simulink model "EV_Modeling"  (R2024b)
(part 5 of 9)

  Signal Specification7/1 -> Divide36/1
  Divide38/1 -> [Motor_Power]
  Constant11/1 -> Switch1/3
  Integrator8/1 -> Position[m]/1, [Current_Position]
  Signal Specification8/1 -> Unit Conversion4/1
  From Workspace18/1 -> Divide33/2
  Add4/1 -> Gain17/1
  " Normalization"/3(Current_n) -> Mux2/3
  Divide22/1 -> Add15/2  "F_friction"
  Zero-Order Hold1/1 -> Extended Kalman Filter/2
  Mux2/1 -> LSTM/1(sequenceinput)
  Divide27/1 -> Add10/1  "Motor_Torque[N.m]"
  " Normalization"/1(Temperature_n) -> Mux2/1
  Divide12/1 -> Add4/1  "Motor_Current"
  Divide11/1 -> Add4/2  "electric_consumption_Current"
  Zero-Order Hold/1 -> Extended Kalman Filter/1
  Extended Kalman Filter/1 -> Gain5/1
  Vol_pack/1 -> Divide12/2
  SOC-Vol/1 -> Voltage_cell/1, " Normalization"/2(Voltage), Vol-R/1, Divide11/1, Vol_pack/1  "Vsoc"
  Coulomb Counting/1(SOC_CC) -> SOC switch/3, Zero-Order Hold/1
  Gain5/1 -> Battery_SOC[%]/1, SOC switch/1  "LSTM_FV2"
  " Normalization"/2(Voltage_n) -> Mux2/2
  MAX Torque1/1 -> Divide27/2, Divide20/1
  Constant10/1 -> Divide35/2
  SOC_t-1/1 -> SOC-Vol/1, SOC-Temp/1
  [Electric_Power] -> Divide12/1
  [Motor_Power] -> Divide39/1
  SOC-Temp/1 -> Temperature_cell/1, " Normalization"/1(Temperature)
  Vol-R/1 -> Divide11/2
  [Motor_RPM] -> MAX Torque1/1
  Constant8/1 -> Add13/1
  Gain17/1 -> Current_cell/1, " Normalization"/3(Current), Coulomb Counting/1(Motor_Current_cell)  "Motor_Current_cell"
  Gain14/1 -> BPP[%]*MAX_Brake_Force[N]1/1
  LSTM/1(SOC) -> Zero-Order Hold1/1  "predictedSOC"
  Unit Conversion3/1 -> Signal Specification7/1
  SOC switch/1 -> SOC_t-1/1
  [T_motor] -> Divide38/1
  Gain20/1 -> [Motor_RPM]
  Step/1 -> SOC switch/2
  connections:
  Simulink-PS Converter/RConn1 -- Subsystem/LConn1
